simulink model "ex6"  (Simulink 8.5)
settings: Solver=ode3  StartTime=0.0  StopTime=60  FixedStep=0.001  RelTol=1e-3
settings Model: Creator=Dinis  LastModifiedBy=Dinis  CovModelRefEnable=off
settings DataIOCC: LimitDataPoints=off  SaveFormat=Dataset  SignalLoggingSaveFormat=Dataset
settings OptimizationCC: ExpressionDepthLimit=128
settings DebuggingCC: UnderspecifiedInitializationDetection=Simplified  MergeDetectMultiDrivingBlocksExec=error  FcnCallInpInsideContextMsg=EnableAllAsError  StateNameClashWarn=none
settings HardwareCC: ProdBitPerPointer=64  ProdLargestAtomicFloat=Float  ProdIntDivRoundTo=Zero  ProdEndianess=LittleEndian  ProdHWDeviceType=Specified
settings ModelReferenceCC: PropagateSignalLabelsOutOfModel=on
settings GRTTargetCC: CombineOutputUpdateFcns=on  GRTInterface=off

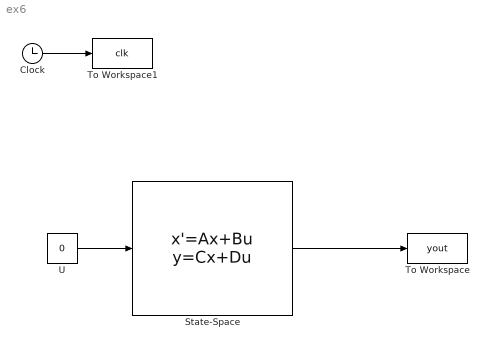
== system ex6 ==
  Clock : Clock
  State-Space : StateSpace  A=[0 1;-45.5802 -0.3749]  B=[0;374.896]  C=[1 0;0 1]  D=[0;0]  X0=[pi/4;0]
  To Workspace : ToWorkspace  VariableName=yout  SaveFormat=Structure With Time  SampleTime=-1
  To Workspace1 : ToWorkspace  VariableName=clk  SampleTime=-1
  U : Constant  Value=0
  wires:
  State-Space/1 -> To Workspace/1
  Clock/1 -> To Workspace1/1
  U/1 -> State-Space/1
